simulink model "Gesamtmodell_Test"  (R2020a)
settings: Solver=VariableStepAuto  StartTime=0.0  StopTime=30  MaxStep=0.01  RelTol=1e-3
settings Model: Creator=Tobias  LastModifiedBy=Frederik
settings SolverCC: ZeroCrossAlgorithm=Adaptive
settings DebuggingCC: IgnoredZcDiagnostic=none

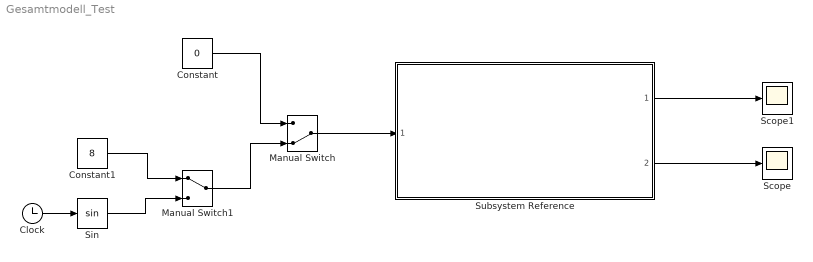
== system Gesamtmodell_Test ==
  Clock : Clock
  Constant : Constant  Value=0
  Constant1 : Constant  Value=8
  Manual Switch : ManualSwitch  CurrentSetting=0
  Manual Switch1 : ManualSwitch
  Scope : Scope
  Scope1 : Scope
  Sin : Trigonometry
  Subsystem Reference : Subsystem  ReferencedSubsystem=Gesamtmodell  ModellParameter=simparams.gesamtmodell
  wires:
  Constant/1 -> Manual Switch/1
  Subsystem Reference/2 -> Scope/1
  Subsystem Reference/1 -> Scope1/1
  Manual Switch/1 -> Subsystem Reference/1
  Manual Switch1/1 -> Manual Switch/2
  Constant1/1 -> Manual Switch1/1
  Sin/1 -> Manual Switch1/2
  Clock/1 -> Sin/1
